simulink model "system_EKF_rendes_ACEKF_validation"  (R2020b)
settings: Solver=VariableStepAuto  StartTime=0.0  StopTime=2  RelTol=1e-3
values from neighbouring files (symbols this model uses):
  e1_noise_std = 0.05    [system_EKF_rendes_ws.m]
  e2_noise_std = deg2rad(0.5)    [system_EKF_rendes_ws.m]
  P0 = eye(4) * 1000    [system_EKF_rendes_ws.m]
  Q = Q_e1 + Q_e2    [system_EKF_rendes_ws.m]
  R = diag([5^2, 10^2])    [system_EKF_rendes_ws.m]
  T = 0.01    [ode_try.m]    (also in system_EKF_rendes_ws.m)
  treshold = 1    [system_EKF_rendes_ws.m]
  vehicleParams = struct('Cf', Cf, 'Cr', Cr, 'lf', lf, 'lr', lr, 'm', m, 'Iz', Iz)    [system_EKF_rendes_ws.m]
  x0 = x_Prior    [ode_try.m]    (also in system_EKF_rendes_ws.m = zeros(4, 1))
settings Model: Creator=Lindenmaier  LastModifiedBy=Admin

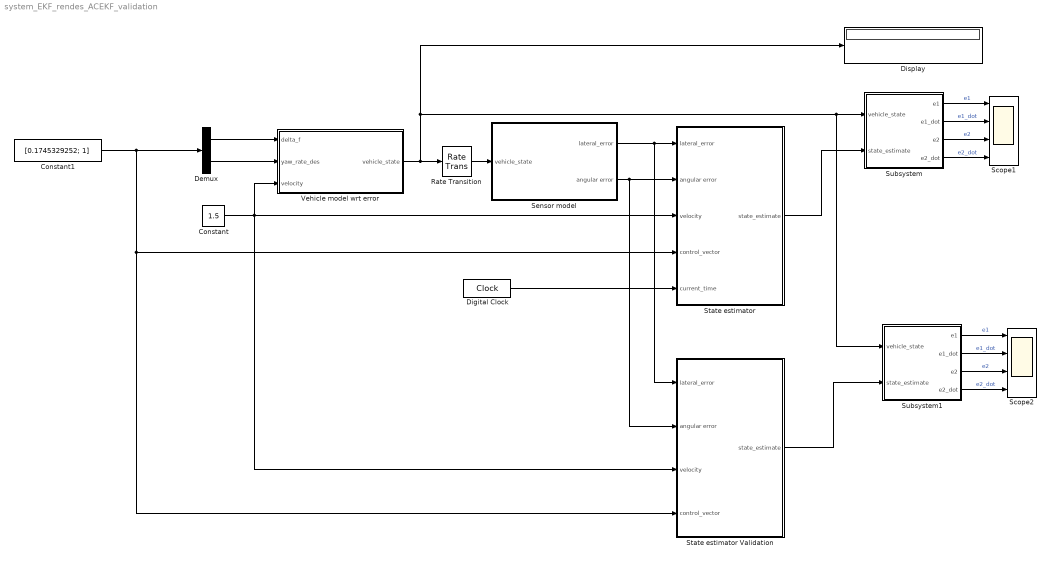
== system system_EKF_rendes_ACEKF_validation ==
  Constant : Constant  Value=1.5
  Constant1 : Constant  Value=[0.1745329252; 1]
  Demux : Demux  Outputs=2
  Digital Clock : DigitalClock  SampleTime=T
  Display : Display
  Rate Transition : RateTransition  OutPortSampleTime=T
  Scope1 : Scope  NumInputPorts=4
  Scope2 : Scope  NumInputPorts=4
  Sensor model : Subsystem
  State estimator : Subsystem
  State estimator Validation : Subsystem
  Subsystem : Subsystem
  Subsystem1 : Subsystem
  Vehicle model wrt error : Subsystem
  wires:
  Vehicle model wrt error/1(vehicle_state) -> Display/1, Subsystem1/1(vehicle_state), Subsystem/1(vehicle_state), Rate Transition/1
  Rate Transition/1 -> Sensor model/1(vehicle_state)
  Sensor model/1(lateral_error) -> State estimator Validation/1(lateral_error), State estimator/1(lateral_error)
  Sensor model/2(angular error) -> State estimator Validation/2(angular error), State estimator/2(angular error)
  Constant/1 -> State estimator Validation/3(velocity), State estimator/3(velocity), Vehicle model wrt error/3(velocity)
  Constant1/1 -> State estimator Validation/4(control_vector), State estimator/4(control_vector), Demux/1
  Demux/1 -> Vehicle model wrt error/1(delta_f)
  Demux/2 -> Vehicle model wrt error/2(yaw_rate_des)
  State estimator/1(state_estimate) -> Subsystem/2(state_estimate)
  Subsystem/1(e1) -> Scope1/1  "e1"
  Subsystem/2(e1_dot) -> Scope1/2  "e1_dot"
  Subsystem/3(e2) -> Scope1/3  "e2"
  Subsystem/4(e2_dot) -> Scope1/4  "e2_dot"
  Digital Clock/1 -> State estimator/5(current_time)
  Subsystem1/4(e2_dot) -> Scope2/4  "e2_dot"
  Subsystem1/3(e2) -> Scope2/3  "e2"
  Subsystem1/2(e1_dot) -> Scope2/2  "e1_dot"
  Subsystem1/1(e1) -> Scope2/1  "e1"
  State estimator Validation/1(state_estimate) -> Subsystem1/2(state_estimate)

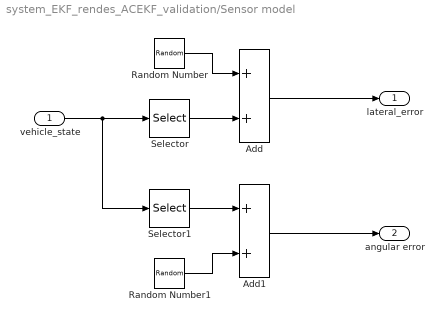
== system system_EKF_rendes_ACEKF_validation/Sensor model ==
  vehicle_state : Inport
  Add : Sum
  Add1 : Sum
  Random Number : RandomNumber  Variance=e1_noise_std^2  SampleTime=T
  Random Number1 : RandomNumber  Variance=e2_noise_std^2  Seed=1  SampleTime=T
  Selector : Selector  InputPortWidth=4  IndexOptions=Index vector (dialog)  Indices=1  OutputSizes=1
  Selector1 : Selector  InputPortWidth=4  IndexOptions=Index vector (dialog)  Indices=3  OutputSizes=1
  lateral_error : Outport
  angular error : Outport  Port=2
  wires:
  vehicle_state/1 -> Selector1/1, Selector/1
  Selector/1 -> Add/2
  Random Number/1 -> Add/1
  Selector1/1 -> Add1/1
  Random Number1/1 -> Add1/2
  Add/1 -> lateral_error/1
  Add1/1 -> angular error/1

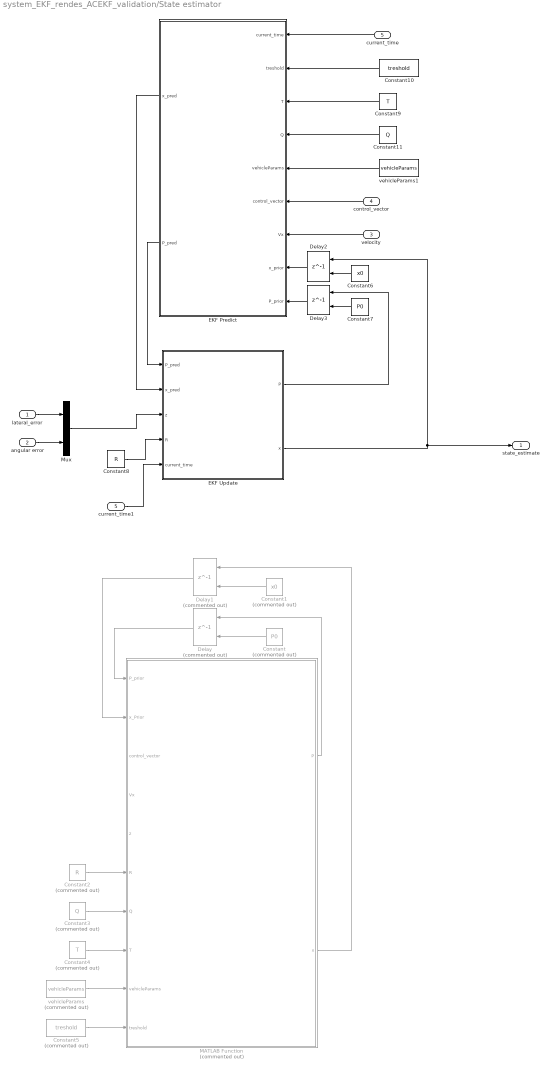
== system system_EKF_rendes_ACEKF_validation/State estimator ==
  lateral_error : Inport
  angular error : Inport  Port=2
  velocity : Inport  Port=3
  control_vector : Inport  Port=4
  current_time : Inport  Port=5
  Constant : Constant  Commented=on  Value=P0
  Constant1 : Constant  Commented=on  Value=x0
  Constant10 : Constant  Value=treshold
  Constant11 : Constant  Value=Q
  Constant2 : Constant  Commented=on  Value=R
  Constant3 : Constant  Commented=on  Value=Q
  Constant4 : Constant  Commented=on  Value=T
  Constant5 : Constant  Commented=on  Value=treshold
  Constant6 : Constant  Value=x0
  Constant7 : Constant  Value=P0
  Constant8 : Constant  Value=R
  Constant9 : Constant  Value=T
  Delay : Delay  Commented=on  DelayLength=1  InitialConditionSource=Input port
      settings: InputPortMap=u0,p4
  Delay1 : Delay  Commented=on  DelayLength=1  InitialConditionSource=Input port
      settings: InputPortMap=u0,p4
  Delay2 : Delay  DelayLength=1  InitialConditionSource=Input port  SampleTime=T
      settings: InputPortMap=u0,p4
  Delay3 : Delay  DelayLength=1  InitialConditionSource=Input port  SampleTime=T
      settings: InputPortMap=u0,p4
  EKF Predict : MATLAB Function  TreatAsAtomicUnit=on
  EKF Update : MATLAB Function  TreatAsAtomicUnit=on
  MATLAB Function : MATLAB Function  Commented=on  TreatAsAtomicUnit=on
  Mux : Mux  Inputs=2
  current_time1 : InportShadow  Port=5
  vehicleParams : Constant  Commented=on  Value=vehicleParams  OutDataTypeStr=Bus: vehicleParamsBus
  vehicleParams1 : Constant  Value=vehicleParams  OutDataTypeStr=Bus: vehicleParamsBus
  state_estimate : Outport
  wires:
  lateral_error/1 -> Mux/1
  angular error/1 -> Mux/2
  EKF Update/2(x) -> Delay2/1, state_estimate/1
  EKF Predict/1(x_pred) -> EKF Update/2(x_pred)
  EKF Predict/2(P_pred) -> EKF Update/1(P_pred)
  EKF Update/1(P) -> Delay3/1
  Delay2/1 -> EKF Predict/8(x_prior)
  MATLAB Function/2(x) -> Delay1/1
  MATLAB Function/1(P) -> Delay/1
  Delay/1 -> MATLAB Function/1(P_prior)
  Delay1/1 -> MATLAB Function/2(x_Prior)
  Constant/1 -> Delay/2
  Constant1/1 -> Delay1/2
  Constant2/1 -> MATLAB Function/6(R)
  Constant3/1 -> MATLAB Function/7(Q)
  vehicleParams/1 -> MATLAB Function/9(vehicleParams)
  Constant4/1 -> MATLAB Function/8(T)
  Constant5/1 -> MATLAB Function/10(treshold)
  Constant6/1 -> Delay2/2
  Delay3/1 -> EKF Predict/9(P_prior)
  Constant7/1 -> Delay3/2
  Mux/1 -> EKF Update/3(z)
  velocity/1 -> EKF Predict/7(Vx)
  control_vector/1 -> EKF Predict/6(control_vector)
  vehicleParams1/1 -> EKF Predict/5(vehicleParams)
  Constant8/1 -> EKF Update/4(R)
  Constant9/1 -> EKF Predict/3(T)
  Constant10/1 -> EKF Predict/2(treshold)
  Constant11/1 -> EKF Predict/4(Q)
  current_time/1 -> EKF Predict/1(current_time)
  current_time1/1 -> EKF Update/5(current_time)

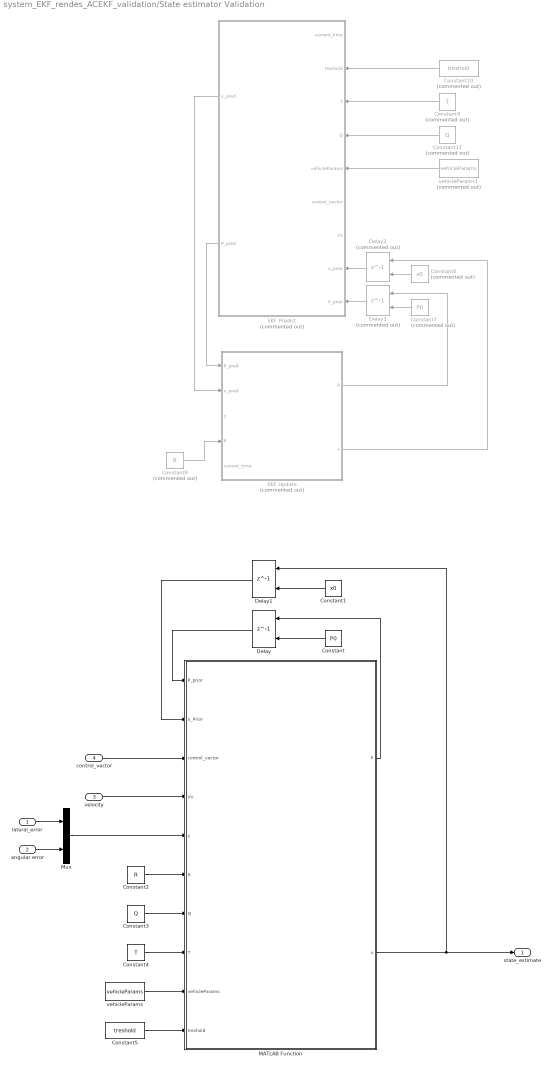
== system system_EKF_rendes_ACEKF_validation/State estimator Validation ==
  lateral_error : Inport
  angular error : Inport  Port=2
  velocity : Inport  Port=3
  control_vector : Inport  Port=4
  Constant : Constant  Value=P0
  Constant1 : Constant  Value=x0
  Constant10 : Constant  Commented=on  Value=treshold
  Constant11 : Constant  Commented=on  Value=Q
  Constant2 : Constant  Value=R
  Constant3 : Constant  Value=Q
  Constant4 : Constant  Value=T
  Constant5 : Constant  Value=treshold
  Constant6 : Constant  Commented=on  Value=x0
  Constant7 : Constant  Commented=on  Value=P0
  Constant8 : Constant  Commented=on  Value=R
  Constant9 : Constant  Commented=on  Value=T
  Delay : Delay  DelayLength=1  InitialConditionSource=Input port
      settings: InputPortMap=u0,p4
  Delay1 : Delay  DelayLength=1  InitialConditionSource=Input port
      settings: InputPortMap=u0,p4
  Delay2 : Delay  Commented=on  DelayLength=1  InitialConditionSource=Input port  SampleTime=T
      settings: InputPortMap=u0,p4
  Delay3 : Delay  Commented=on  DelayLength=1  InitialConditionSource=Input port  SampleTime=T
      settings: InputPortMap=u0,p4
  EKF Predict : MATLAB Function  Commented=on  TreatAsAtomicUnit=on
  EKF Update : MATLAB Function  Commented=on  TreatAsAtomicUnit=on
  MATLAB Function : MATLAB Function  TreatAsAtomicUnit=on
  Mux : Mux  Inputs=2
  vehicleParams : Constant  Value=vehicleParams  OutDataTypeStr=Bus: vehicleParamsBus
  vehicleParams1 : Constant  Commented=on  Value=vehicleParams  OutDataTypeStr=Bus: vehicleParamsBus
  state_estimate : Outport
  wires:
  Constant11/1 -> EKF Predict/4(Q)
  Constant10/1 -> EKF Predict/2(treshold)
  Constant9/1 -> EKF Predict/3(T)
  Constant8/1 -> EKF Update/4(R)
  vehicleParams1/1 -> EKF Predict/5(vehicleParams)
  Constant7/1 -> Delay3/2
  Delay3/1 -> EKF Predict/9(P_prior)
  Constant6/1 -> Delay2/2
  Constant5/1 -> MATLAB Function/10(treshold)
  Constant4/1 -> MATLAB Function/8(T)
  vehicleParams/1 -> MATLAB Function/9(vehicleParams)
  Constant3/1 -> MATLAB Function/7(Q)
  Constant2/1 -> MATLAB Function/6(R)
  Constant1/1 -> Delay1/2
  Constant/1 -> Delay/2
  Delay1/1 -> MATLAB Function/2(x_Prior)
  Delay/1 -> MATLAB Function/1(P_prior)
  MATLAB Function/1(P) -> Delay/1
  MATLAB Function/2(x) -> Delay1/1, state_estimate/1
  Delay2/1 -> EKF Predict/8(x_prior)
  EKF Update/1(P) -> Delay3/1
  EKF Predict/2(P_pred) -> EKF Update/1(P_pred)
  EKF Predict/1(x_pred) -> EKF Update/2(x_pred)
  EKF Update/2(x) -> Delay2/1
  angular error/1 -> Mux/2
  lateral_error/1 -> Mux/1
  control_vector/1 -> MATLAB Function/3(control_vector)
  velocity/1 -> MATLAB Function/4(Vx)
  Mux/1 -> MATLAB Function/5(z)

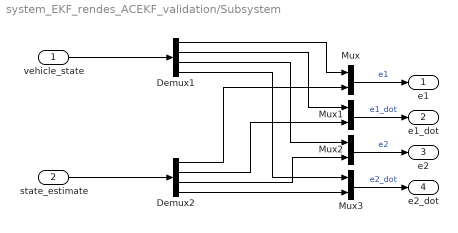
== system system_EKF_rendes_ACEKF_validation/Subsystem ==
  vehicle_state : Inport
  state_estimate : Inport  Port=2
  Demux1 : Demux
  Demux2 : Demux
  Mux{,1..3} (4 alike) : Mux  Inputs=2
  e1 : Outport
  e1_dot : Outport  Port=2
  e2 : Outport  Port=3
  e2_dot : Outport  Port=4
  wires:
  Mux3/1 -> e2_dot/1  "e2_dot"
  Demux2/3 -> Mux2/2
  Demux1/1 -> Mux/1
  Demux2/1 -> Mux/2
  Demux2/2 -> Mux1/2
  Mux/1 -> e1/1  "e1"
  Demux1/2 -> Mux1/1
  Demux1/3 -> Mux2/1
  Demux1/4 -> Mux3/1
  Demux2/4 -> Mux3/2
  vehicle_state/1 -> Demux1/1
  state_estimate/1 -> Demux2/1
  Mux1/1 -> e1_dot/1  "e1_dot"
  Mux2/1 -> e2/1  "e2"

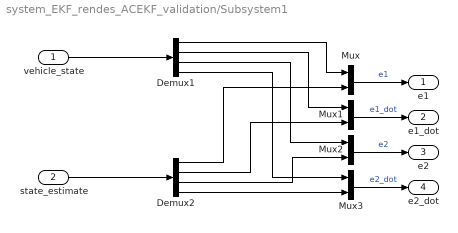
== system system_EKF_rendes_ACEKF_validation/Subsystem1 ==
  vehicle_state : Inport
  state_estimate : Inport  Port=2
  Demux1 : Demux
  Demux2 : Demux
  Mux{,1..3} (4 alike) : Mux  Inputs=2
  e1 : Outport
  e1_dot : Outport  Port=2
  e2 : Outport  Port=3
  e2_dot : Outport  Port=4
  wires:
  Mux2/1 -> e2/1  "e2"
  Mux1/1 -> e1_dot/1  "e1_dot"
  state_estimate/1 -> Demux2/1
  vehicle_state/1 -> Demux1/1
  Demux2/4 -> Mux3/2
  Demux1/4 -> Mux3/1
  Demux1/3 -> Mux2/1
  Demux1/2 -> Mux1/1
  Mux/1 -> e1/1  "e1"
  Demux2/2 -> Mux1/2
  Demux2/1 -> Mux/2
  Demux1/1 -> Mux/1
  Demux2/3 -> Mux2/2
  Mux3/1 -> e2_dot/1  "e2_dot"

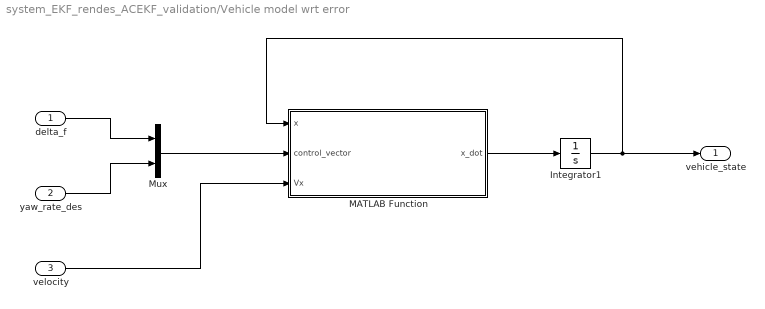
== system system_EKF_rendes_ACEKF_validation/Vehicle model wrt error ==
  delta_f : Inport
  yaw_rate_des : Inport  Port=2
  velocity : Inport  Port=3
  Integrator1 : Integrator
  MATLAB Function : MATLAB Function  TreatAsAtomicUnit=on
  Mux : Mux  Inputs=2
  vehicle_state : Outport
  wires:
  Integrator1/1 -> MATLAB Function/1(x), vehicle_state/1
  yaw_rate_des/1 -> Mux/2
  delta_f/1 -> Mux/1
  MATLAB Function/1(x_dot) -> Integrator1/1
  Mux/1 -> MATLAB Function/2(control_vector)
  velocity/1 -> MATLAB Function/3(Vx)

== matlab function system_EKF_rendes_ACEKF_validation/State estimator Validation/MATLAB Function ==
  data: P_prior input; x_Prior input; control_vector input; P output; Vx input; z input; x output; R input; Q input; T input; vehicleParams input; treshold input
function [P, x] = EKF_predict_update(P_prior, x_Prior, control_vector, Vx, z, R, Q, T, vehicleParams, treshold)

    % Parameters
    Cf = vehicleParams.Cf;
    Cr = vehicleParams.Cr;
    lf = vehicleParams.lf;
    lr = vehicleParams.lr;
    m  = vehicleParams.m;
    Iz = vehicleParams.Iz;

    % State-space model elements
    P1 = -((2*Cf + 2*Cr)/(m * Vx));
    P2 = (2*Cf + 2*Cr) / m;
    P3 = (-2*Cf * lf + 2*Cr * lr) / (m * Vx);
    P4 = -((2*Cf * lf - 2*Cr * lr) / (Iz * Vx));
    P5 = (2*Cf * lf - 2*Cr * lr) / Iz;
    P6 = -((2*Cf * lf^2 + 2*Cr * lr^2) / (Iz * Vx));
    P7 = (2*Cf) / m;
    P8 = -((2*Cf * lf - 2*Cr * lr) / (m * Vx)) - Vx;
    P9 = (2*Cf * lf) / Iz;
    P10 = -(2*Cf * lf^2 + 2*Cr * lr^2) / (Iz * Vx);

    % Continuous-time state-space matrices
    Ac = [0 1 0 0;
          0 P1 P2 P3;
          0 0 0 1;
          0 P4 P5 P6];
      
    Bc = [0 0;
          P7 P8;
          0 0;
          P9 P10];

    Ad = [1.0000    0.0054    0.0069    0.0003;
          0         0.2468    1.1298    0.0230;
          0         0.0004    0.9995    0.0022;
          0         0.0261   -0.0391    0.0117];

    Bd = [0.0038    0.0002;
          0.6280    0.0080;
          0.0034   -0.0078;
          0.4410   -0.9883];
    
    % Discrete-time prediction step 
    x_pred = Ad * x_Prior + Bd * control_vector; 
    P_pred = Ad * P_prior * Ad' + Q;
    
    
    %%%%%%%%%%%%%%%%%%%%%%
    % Update
    % Measurement function (example: measuring only position states)
    h_x = [x_pred(1); x_pred(3)];

    % Calculate Jacobian matrix of h with respect to state
    H = [ 1, 0, 0, 0;
          0, 0, 1, 0];

    % Measurement residual
    y = z - h_x;

    % Innovation covariance
    S = H * P_pred * H' + R;

    % Optimal Kalman gain
    K = P_pred * H' / S;

    % Updated state estimate
    x = x_pred + K * y;

    % Updated estimate covariance
    P = (eye(size(P_pred)) - K * H) * P_pred;


end

== matlab function system_EKF_rendes_ACEKF_validation/State estimator/EKF Predict ==
  data: current_time input; treshold input; T input; Q input; vehicleParams input; control_vector input; Vx input; x_prior input; x_pred output size=[4 1]; P_pred output size=[4 4]; P_prior input
function [x_pred, P_pred] = ekfPredict(current_time, treshold ,T, Q, vehicleParams, control_vector, Vx, x_prior, P_prior)

    % Parameters
    Cf = vehicleParams.Cf;
    Cr = vehicleParams.Cr;
    lf = vehicleParams.lf;
    lr = vehicleParams.lr;
    m  = vehicleParams.m;
    Iz = vehicleParams.Iz;

    % State-space model elements
    P1 = -((2*Cf + 2*Cr)/(m * Vx));
    P2 = (2*Cf + 2*Cr) / m;
    P3 = (-2*Cf * lf + 2*Cr * lr) / (m * Vx);
    P4 = -((2*Cf * lf - 2*Cr * lr) / (Iz * Vx));
    P5 = (2*Cf * lf - 2*Cr * lr) / Iz;
    P6 = -((2*Cf * lf^2 + 2*Cr * lr^2) / (Iz * Vx));
    P7 = (2*Cf) / m;
    P8 = -((2*Cf * lf - 2*Cr * lr) / (m * Vx)) - Vx;
    P9 = (2*Cf * lf) / Iz;
    P10 = -(2*Cf * lf^2 + 2*Cr * lr^2) / (Iz * Vx);

    % Continuous-time state-space matrices
    Ac = [0 1 0 0;
          0 P1 P2 P3;
          0 0 0 1;
          0 P4 P5 P6];
      
    Bc = [0 0;
          P7 P8;
          0 0;
          P9 P10];

    I = eye(4); % Identity matrix

    % Nonlinear state transition function
%     if abs(Vx) < threshold
%         Ad = 
%         Bd = 
%     else
%         Ad = (I + Ac * T);
%         Bd = Bc * T;
%     end
    
    % Discret state
%    Ad = (I + Ac * T);
%    Bd = Bc * T;
    
    % Define the time span for integration
    tspan = [current_time current_time+T]; % Integrate from 0 to T 
    
    % Initial conditions 
    x0 = x_prior; 
    
    % Define input control vector (u)
    u = control_vector;

    % Initialize t and x for clarity 
%     t = []; 
%     x = [];
    
    % Solve the state equation using ode45 
    [~, x_sol] = ode45(@(t, x) Ac*x + Bc*u, tspan, x0);

    
    % Predicted state (x_pred) 
    x_pred = x_sol(end,:)';

    % Calculate Jacobian matrix of f() with respect to x
    F = Ac;
     
     % Calculate FQF
%     q11 = Q(1,1);
%     q22 = Q(2,2);
%     q33 = Q(3,3);
%     q44 = Q(4,4);
%     
%     FQF_11 = q22;
%     FQF_12 = P1*q22;
%     FQF_13 = 0;
%     FQF_14 = P4*q22;
%     FQF_21 = P1*q22;
%     FQF_22 = P1^2*q22+P2^2*q33+P3^2*q44;
%     FQF_23 = 0;
%     FQF_24 = P1*P4*q22 + P2*P5*q33 + P6*P3*q44;
%     FQF_31 = 0;
%     FQF_32 = P3*q44;
%     FQF_33 = 0;
%     FQF_34 = P6*q44;
%     FQF_41 = P4*q22;
%     FQF_42 = P1*P4*q22 + P2*P5*q33 + P3*P6*q44;
%     FQF_43 = 0;
%     FQF_44 = P4^2*q22 + P5^2*q33 + P6^2*q44;
%     
%     FQF = [FQF_11 FQF_12 FQF_13 FQF_14;
%            FQF_21 FQF_22 FQF_23 FQF_24;
%            FQF_31 FQF_32 FQF_33 FQF_34;
%            FQF_41 FQF_42 FQF_43 FQF_44];

    % Time-update (prediction) step
%     x_pred = Ad * x_Prior + Bd * control_vector;
    P_pred = (I + T * F) * P_prior * (I + T * F)' + Q;
    
end

== matlab function system_EKF_rendes_ACEKF_validation/State estimator/EKF Update ==
  data: P output; P_pred input; x_pred input; z input; x output; R input; current_time input
function [P, x] = ekfUpdate(P_pred, x_pred, z, R, current_time)

    % Update
    % Measurement function (example: measuring only position states)
    h_x = [x_pred(1); x_pred(3)];

    % Calculate Jacobian matrix of h with respect to state
    H = [ 1, 0, 0, 0;
          0, 0, 1, 0];

    % Measurement residual
    y = z - h_x;

    % Innovation covariance
    S = H * P_pred * H' + R;

    % Optimal Kalman gain
    K = P_pred * H' / S;

    % Updated state estimate
    x = x_pred + K * y;

    % Updated estimate covariance
    P = (eye(size(P_pred)) - K * H) * P_pred;

end

== matlab function system_EKF_rendes_ACEKF_validation/State estimator Validation/EKF Predict ==
  data: current_time input; treshold input; T input; Q input; vehicleParams input; control_vector input; Vx input; x_prior input; x_pred output size=[4 1]; P_pred output size=[4 4]; P_prior input
function [x_pred, P_pred] = ekfPredict(current_time, treshold ,T, Q, vehicleParams, control_vector, Vx, x_prior, P_prior)

    % Parameters
    Cf = vehicleParams.Cf;
    Cr = vehicleParams.Cr;
    lf = vehicleParams.lf;
    lr = vehicleParams.lr;
    m  = vehicleParams.m;
    Iz = vehicleParams.Iz;

    % State-space model elements
    P1 = -((2*Cf + 2*Cr)/(m * Vx));
    P2 = (2*Cf + 2*Cr) / m;
    P3 = (-2*Cf * lf + 2*Cr * lr) / (m * Vx);
    P4 = -((2*Cf * lf - 2*Cr * lr) / (Iz * Vx));
    P5 = (2*Cf * lf - 2*Cr * lr) / Iz;
    P6 = -((2*Cf * lf^2 + 2*Cr * lr^2) / (Iz * Vx));
    P7 = (2*Cf) / m;
    P8 = -((2*Cf * lf - 2*Cr * lr) / (m * Vx)) - Vx;
    P9 = (2*Cf * lf) / Iz;
    P10 = -(2*Cf * lf^2 + 2*Cr * lr^2) / (Iz * Vx);

    % Continuous-time state-space matrices
    Ac = [0 1 0 0;
          0 P1 P2 P3;
          0 0 0 1;
          0 P4 P5 P6];
      
    Bc = [0 0;
          P7 P8;
          0 0;
          P9 P10];

    I = eye(4); % Identity matrix

    % Nonlinear state transition function
%     if abs(Vx) < threshold
%         Ad = 
%         Bd = 
%     else
%         Ad = (I + Ac * T);
%         Bd = Bc * T;
%     end
    
    % Discret state
%    Ad = (I + Ac * T);
%    Bd = Bc * T;
    
    % Define the time span for integration
    tspan = [current_time current_time+T]; % Integrate from 0 to T 
    
    % Initial conditions 
    x0 = x_prior; 
    
    % Define input control vector (u)
    u = control_vector;

    % Initialize t and x for clarity 
%     t = []; 
%     x = [];
    
    % Solve the state equation using ode45 
    [~, x_sol] = ode45(@(t, x) Ac*x + Bc*u, tspan, x0);

    
    % Predicted state (x_pred) 
    x_pred = x_sol(end,:)';

    % Calculate Jacobian matrix of f() with respect to x
    F = Ac;
     
     % Calculate FQF
%     q11 = Q(1,1);
%     q22 = Q(2,2);
%     q33 = Q(3,3);
%     q44 = Q(4,4);
%     
%     FQF_11 = q22;
%     FQF_12 = P1*q22;
%     FQF_13 = 0;
%     FQF_14 = P4*q22;
%     FQF_21 = P1*q22;
%     FQF_22 = P1^2*q22+P2^2*q33+P3^2*q44;
%     FQF_23 = 0;
%     FQF_24 = P1*P4*q22 + P2*P5*q33 + P6*P3*q44;
%     FQF_31 = 0;
%     FQF_32 = P3*q44;
%     FQF_33 = 0;
%     FQF_34 = P6*q44;
%     FQF_41 = P4*q22;
%     FQF_42 = P1*P4*q22 + P2*P5*q33 + P3*P6*q44;
%     FQF_43 = 0;
%     FQF_44 = P4^2*q22 + P5^2*q33 + P6^2*q44;
%     
%     FQF = [FQF_11 FQF_12 FQF_13 FQF_14;
%            FQF_21 FQF_22 FQF_23 FQF_24;
%            FQF_31 FQF_32 FQF_33 FQF_34;
%            FQF_41 FQF_42 FQF_43 FQF_44];

    % Time-update (prediction) step
%     x_pred = Ad * x_Prior + Bd * control_vector;
    P_pred = (I + T * F) * P_prior * (I + T * F)' + Q;
    
end

== matlab function system_EKF_rendes_ACEKF_validation/Vehicle model wrt error/MATLAB Function ==
  data: x input; x_dot output; control_vector input; Vx input
function x_dot = countinous_model(x, control_vector, Vx)

    % Parameters
    Cf=80000;
    Cr=80000;
    lf=1.4;
    lr=1.8;
    m=1500;
    Iz=1200;

    % Elements
    P1 = -((2*Cf+2*Cr)/(m*Vx));
    P2 = (2*Cf+2*Cr)/m;
    P3 = (-2*Cf*lf+2*Cr*lr)/(m*Vx);
    P4 = -((2*Cf*lf-2*Cr*lr)/(Iz*Vx));
    P5 = (2*Cf*lf-2*Cr*lr)/Iz;
    P6 = -((2*Cf*lf^2+2*Cr*lr^2)/(Iz*Vx));
    P7 = (2*Cf)/m;
    P8 = -((2*Cf*lf-2*Cr*lr)/(m*Vx))-Vx;
    P9 = (2*Cf*lf)/Iz;
    P10 = -(2*Cf*lf^2+2*Cr*lr^2)/(Iz*Vx);

    % State space
    Ac=[0 1  0  0;
        0 P1 P2 P3;
        0 0  0  1;
        0 P4 P5 P6]; 

    Bc=[0  0;
        P7 P8;
        0  0;
        P9 P10];
                  
x_dot = Ac*x + Bc*control_vector;

== matlab function system_EKF_rendes_ACEKF_validation/State estimator/MATLAB Function ==
  data: P_prior input; x_Prior input; control_vector input; P output; Vx input; z input; x output; R input; Q input; T input; vehicleParams input; treshold input
function [P, x] = EKF_predict_update(P_prior, x_Prior, control_vector, Vx, z, R, Q, T, vehicleParams, treshold)

    % Parameters
    Cf = vehicleParams.Cf;
    Cr = vehicleParams.Cr;
    lf = vehicleParams.lf;
    lr = vehicleParams.lr;
    m  = vehicleParams.m;
    Iz = vehicleParams.Iz;

    % State-space model elements
    P1 = -((2*Cf + 2*Cr)/(m * Vx));
    P2 = (2*Cf + 2*Cr) / m;
    P3 = (-2*Cf * lf + 2*Cr * lr) / (m * Vx);
    P4 = -((2*Cf * lf - 2*Cr * lr) / (Iz * Vx));
    P5 = (2*Cf * lf - 2*Cr * lr) / Iz;
    P6 = -((2*Cf * lf^2 + 2*Cr * lr^2) / (Iz * Vx));
    P7 = (2*Cf) / m;
    P8 = -((2*Cf * lf - 2*Cr * lr) / (m * Vx)) - Vx;
    P9 = (2*Cf * lf) / Iz;
    P10 = -(2*Cf * lf^2 + 2*Cr * lr^2) / (Iz * Vx);

    % Continuous-time state-space matrices
    Ac = [0 1 0 0;
          0 P1 P2 P3;
          0 0 0 1;
          0 P4 P5 P6];
      
    Bc = [0 0;
          P7 P8;
          0 0;
          P9 P10];

    I = eye(4); % Identity matrix

    % Nonlinear state transition function
%     if abs(Vx) < threshold
%         Ad = 
%         Bd = 
%     else
%         Ad = (I + Ac * T);
%         Bd = Bc * T;
%     end
    
    Ad = (I + Ac * T);
    Bd = Bc * T;
    
    % Calculate Jacobian matrix of f() with respect to x
    F = [1 T      0    0;
         0 1+P1*T P2*T P3*T;
         0 0      0    1;
         0 P4*T   P5*T 1+P6*T];

%     F = Ac;
     
    % Calculate Qk
    q11 = Q(1,1);
    q22 = Q(2,2);
    q33 = Q(3,3);
    q44 = Q(4,4);
    
    Qk_11 = (T^3/3)*q22 + T*q11;
    Qk_12 = ((T^3/3)*P1 + (T^2/2))*q22;
    Qk_13 = 0;
    Qk_14 = (T^3/3)*P4*q22;
    Qk_21 = (T^2/2 + (T^3/3)*P1)*q22;
    Qk_22 = ((1+P1*T)^3/(3*P1))*q22 + (T^3/3)*P2*q33 + (T^3/3)*P3*q44;
    Qk_23 = (T^3/3)*P3*q44 + (T^2/2)*P2*q33;
    Qk_24 = (T^2/2+(T^3/3)*P1)*P4*q22 + (T^2/2+(T^3/3)*P6)*P3*q44 + (T^3/3)*P2*P5*q33;
    Qk_31 = 0;
    Qk_32 = (T^3/3)*P3*q44 + (T^2/2)*P2*q33;
    Qk_33 = (T^3/3)*q44 + T*q33;
    Qk_34 = (T^2/2)*P5*q33 + ((T^3/3)*P6+T^2/2)*q44;
    Qk_41 = (T^3/3)*P4*q22;
    Qk_42 = (T^2/2+(T^3/3)*P1)*P4*q22 + (T^2/2+(T^3/3)*P6)*P3*q44 + (T^3/3)*P2*P5*q33;
    Qk_43 = (T^2/2+(T^3/3)*P6)*q44 + (T^2/2)*P5*q33;
    Qk_44 = ((1+P6*T)^3/(3*P6))*q44 + (T^3/3)*P4*q22 + (T^3/3)*P5*q33;
    
    Qk = [Qk_11 Qk_12 Qk_13 Qk_14;
          Qk_21 Qk_22 Qk_23 Qk_24;
          Qk_31 Qk_32 Qk_33 Qk_34;
          Qk_41 Qk_42 Qk_43 Qk_44];

    % Time-update (prediction) step
    x_pred = Ad * x_Prior + Bd * control_vector;
    P_pred = (I + T * F) * P_prior * (I + T * F)' + Q*T;
%     P_pred = F * P_prior * F' + Qk;
    
    
    %%%%%%%%%%%%%%%%%%%%%%
    % Update
    % Measurement function (example: measuring only position states)
    h_x = [x_pred(1); x_pred(3)];

    % Calculate Jacobian matrix of h with respect to state
    H = [ 1, 0, 0, 0;
          0, 0, 1, 0];

    % Measurement residual
    y = z - h_x;

    % Innovation covariance
    S = H * P_pred * H' + R;

    % Optimal Kalman gain
    K = P_pred * H' / S;

    % Updated state estimate
    x = x_pred + K * y;

    % Updated estimate covariance
    P = (eye(size(P_pred)) - K * H) * P_pred;


end

== matlab function system_EKF_rendes_ACEKF_validation/State estimator Validation/EKF Update ==
  data: P output; P_pred input; x_pred input; z input; x output; R input; current_time input
function [P, x] = ekfUpdate(P_pred, x_pred, z, R, current_time)

    % Update
    % Measurement function (example: measuring only position states)
    h_x = [x_pred(1); x_pred(3)];

    % Calculate Jacobian matrix of h with respect to state
    H = [ 1, 0, 0, 0;
          0, 0, 1, 0];

    % Measurement residual
    y = z - h_x;

    % Innovation covariance
    S = H * P_pred * H' + R;

    % Optimal Kalman gain
    K = P_pred * H' / S;

    % Updated state estimate
    x = x_pred + K * y;

    % Updated estimate covariance
    P = (eye(size(P_pred)) - K * H) * P_pred;

end
